simulink model "estimator_ICE8"  (R2023a)
settings: Solver=ode45  StartTime=0.0  StopTime=6  RelTol=1e-3  EnableMultiTasking=on
undefined symbols (not defined in the file): A, ahat, B, C, G_fast, xhat0
settings Model: Creator=kiriakid  LastModifiedBy=m260477
settings SolverCC: AlgebraicLoopSolver=TrustRegion
settings DataIOCC: SaveFormat=Array  SignalLoggingSaveFormat=ModelDataLogs  ReturnWorkspaceOutputs=off
settings OptimizationCC: BlockReduction=off  BooleanDataType=off  ExpressionDepthLimit=2147483647  InitFltsAndDblsToZero=on  LifeSpan=inf
settings DebuggingCC: SaveWithParameterizedLinksMsg=none  UnderspecifiedInitializationDetection=Classic  MergeDetectMultiDrivingBlocksExec=none  SignalResolutionControl=TryResolveAllWithWarning  MultiTaskDSMMsg=warning  MultiTaskCondExecSysMsg=none  FcnCallInpInsideContextMsg=warning  UnconnectedInputMsg=warning  UnconnectedOutputMsg=warning  UnconnectedLineMsg=warning  StateNameClashWarn=warning  SFUnexpectedBacktrackingDiag=warning  SFNoUnconditionalDefaultTransitionDiag=warning  SFExecutionAtInitializationDiag=none  ArithmeticOperatorsInVariantConditions=warning
settings HardwareCC: ProdBitPerPointer=32  ProdBitPerSizeT=32  ProdBitPerPtrDiffT=32  ProdLargestAtomicFloat=None  ProdIntDivRoundTo=Undefined  ProdEndianess=Unspecified  ProdWordSize=32  ProdHWDeviceType=32-bit Generic  TargetUnknown=on
settings ModelReferenceCC: EnableRefExpFcnMdlSchedulingChecks=on  PropagateSignalLabelsOutOfModel=off
settings SFSimCC: SimUseLocalCustomCode=off  CustomCodeUndefinedFunction=UseInterfaceOnly
settings RTWCC: RTWUseLocalCustomCode=off
settings CodeAppCC: StateflowObjectComments=on
settings GRTTargetCC: TargetFcnLib=ansi_tfl_tmw.mat  TargetLangStandard=C89/C90 (ANSI)  CombineOutputUpdateFcns=off  GRTInterface=on
settings ConfigComp: CovMetricSettings=dw  CovSaveCumulativeToWorkspaceVar=on  CovSaveSingleToWorkspaceVar=on  CovExternalEMLEnable=off

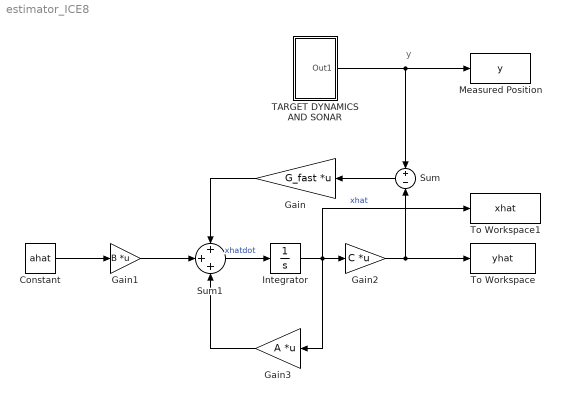
== system estimator_ICE8 ==
  note: y
  Constant : Constant  Value=ahat
  Gain : Gain  Gain=G_fast  Multiplication=Matrix(K*u)
  Gain1 : Gain  Gain=B  Multiplication=Matrix(K*u)
  Gain2 : Gain  Gain=C  Multiplication=Matrix(K*u)
  Gain3 : Gain  Gain=A  Multiplication=Matrix(K*u)
  Integrator : Integrator  InitialCondition=xhat0
  Measured Position : ToWorkspace  VariableName=y  SampleTime=-1
      settings: Save2DSignal=2-D array (concatenate along first dimension)
  Sum : Sum  Inputs=+|-
  Sum1 : Sum  Inputs=+++
  TARGET DYNAMICS AND SONAR : Subsystem
  To Workspace : ToWorkspace  VariableName=yhat  SampleTime=-1
  To Workspace1 : ToWorkspace  VariableName=xhat  SampleTime=-1
  wires:
  TARGET DYNAMICS AND SONAR/1(Out1) -> Measured Position/1, Sum/1
  Sum/1 -> Gain/1
  Gain1/1 -> Sum1/2
  Gain/1 -> Sum1/1
  Sum1/1 -> Integrator/1  "xhatdot"
  Gain2/1 -> Sum/2, To Workspace/1
  Integrator/1 -> To Workspace1/1, Gain3/1, Gain2/1  "xhat"
  Gain3/1 -> Sum1/3
  Constant/1 -> Gain1/1

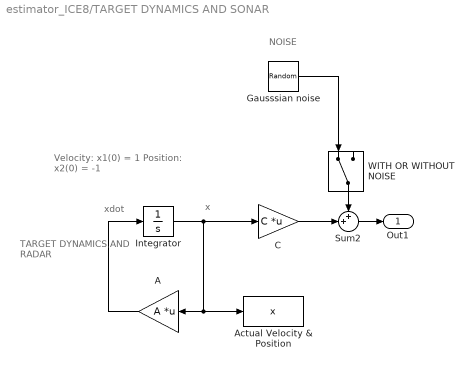
== system estimator_ICE8/TARGET DYNAMICS AND SONAR ==
  note: NOISE
  note: TARGET
      |  DYNAMICS
      | AND
      | RADAR
  note: x
  note: xdot
  note: Velocity:  x1(0) = 1
      | Position:  x2(0) = -1
  A : Gain  Gain=A  Multiplication=Matrix(K*u)  SaturateOnIntegerOverflow=on  OutDataTypeStr=Inherit: Same as input  ParamDataTypeStr=Inherit: Same as input
  Actual Velocity & Position : ToWorkspace  VariableName=x  SampleTime=-1
  C : Gain  Gain=C  Multiplication=Matrix(K*u)  SaturateOnIntegerOverflow=on  OutDataTypeStr=Inherit: Same as input  ParamDataTypeStr=Inherit: Same as input
  Gausssian noise : RandomNumber  Variance=0.005  SampleTime=0.001
  Integrator : Integrator  InitialCondition=[1 -1]
  Sum2 : Sum  Inputs=++|  InputSameDT=on  SaturateOnIntegerOverflow=on  OutDataTypeStr=Inherit: Same as first input
  WITH OR WITHOUT NOISE : ManualSwitch
  Out1 : Outport  VectorParamsAs1DForOutWhenUnconnected=off
  wires:
  WITH OR WITHOUT NOISE/1 -> Sum2/1
  C/1 -> Sum2/2
  A/1 -> Integrator/1
  Integrator/1 -> C/1, A/1, Actual Velocity & Position/1
  Sum2/1 -> Out1/1
  Gausssian noise/1 -> WITH OR WITHOUT NOISE/1
